simulink library "multi_sensor_dynamics"  (R2021a)
settings: Solver=VariableStepAuto  StartTime=0.0  StopTime=10.0  RelTol=1e-3
undefined symbols (not defined in the file): config
libraries: attitude_library x5, vrlib x3
settings Model: Creator=Laura  LastModifiedBy=Laura

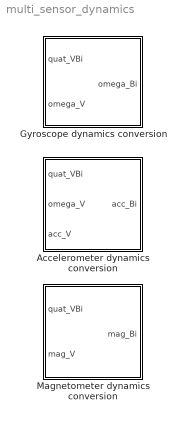
== system multi_sensor_dynamics ==
  Accelerometer dynamics conversion : Subsystem
  Gyroscope dynamics conversion : Subsystem
  Magnetometer dynamics conversion : Subsystem

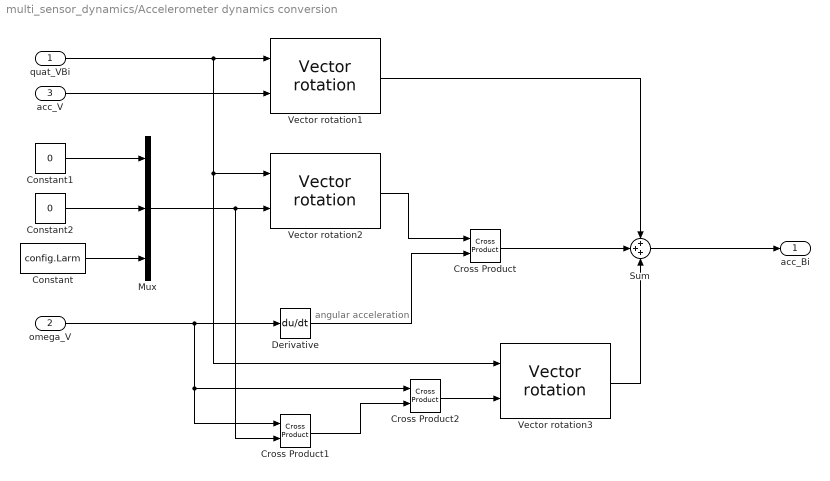
== system multi_sensor_dynamics/Accelerometer dynamics conversion ==
  note: angular acceleration
  quat_VBi : Inport
  omega_V : Inport  Port=2
  acc_V : Inport  Port=3
  Constant : Constant  Value=config.Larm
  Constant1 : Constant  Value=0
  Constant2 : Constant  Value=0
  Cross Product : vrlib/Utilities/Cross Product
  Cross Product1 : vrlib/Utilities/Cross Product
  Cross Product2 : vrlib/Utilities/Cross Product
  Derivative : Derivative
  Mux : Mux  Inputs=3
  Sum : Sum  Inputs=+++
  Vector rotation1 : attitude_library/Vector rotation  SystemSampleTime=-1  VariantActivationTime=update diagram  Latency=0  AutoFrameSizeCalculation=off
  Vector rotation2 : attitude_library/Vector rotation  SystemSampleTime=-1  VariantActivationTime=update diagram  Latency=0  AutoFrameSizeCalculation=off
  Vector rotation3 : attitude_library/Vector rotation  SystemSampleTime=-1  VariantActivationTime=update diagram  Latency=0  AutoFrameSizeCalculation=off
  acc_Bi : Outport
  wires:
  omega_V/1 -> Cross Product2/1, Cross Product1/1, Derivative/1
  quat_VBi/1 -> Vector rotation3/1, Vector rotation2/1, Vector rotation1/1
  acc_V/1 -> Vector rotation1/2
  Vector rotation1/1 -> Sum/1
  Constant1/1 -> Mux/1
  Constant2/1 -> Mux/2
  Constant/1 -> Mux/3
  Mux/1 -> Cross Product1/2, Vector rotation2/2
  Cross Product/1 -> Sum/2
  Vector rotation2/1 -> Cross Product/1
  Derivative/1 -> Cross Product/2
  Sum/1 -> acc_Bi/1
  Cross Product1/1 -> Cross Product2/2
  Vector rotation3/1 -> Sum/3
  Cross Product2/1 -> Vector rotation3/2

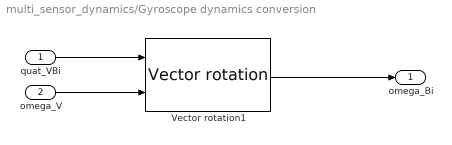
== system multi_sensor_dynamics/Gyroscope dynamics conversion ==
  quat_VBi : Inport
  omega_V : Inport  Port=2
  Vector rotation1 : attitude_library/Vector rotation  SystemSampleTime=-1  VariantActivationTime=update diagram  Latency=0  AutoFrameSizeCalculation=off
  omega_Bi : Outport
  wires:
  Vector rotation1/1 -> omega_Bi/1
  quat_VBi/1 -> Vector rotation1/1
  omega_V/1 -> Vector rotation1/2

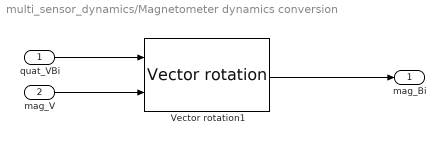
== system multi_sensor_dynamics/Magnetometer dynamics conversion ==
  quat_VBi : Inport
  mag_V : Inport  Port=2
  Vector rotation1 : attitude_library/Vector rotation  SystemSampleTime=-1  VariantActivationTime=update diagram  Latency=0  AutoFrameSizeCalculation=off
  mag_Bi : Outport
  wires:
  quat_VBi/1 -> Vector rotation1/1
  mag_V/1 -> Vector rotation1/2
  Vector rotation1/1 -> mag_Bi/1
